simulink model "CIP_LQR_Servo"  (R2022b)
settings: Solver=ode1  StartTime=0.0  StopTime=10  FixedStep=1/1000  MaxStep=0.01  RelTol=1e-3  EnableMultiTasking=on
values from neighbouring files (symbols this model uses):
  b = [x(3) ... (first row only)    [f_inv_cart_pend.m]    (also in m_CIP_LQR_Servo.m = 0.5)
  c = 0.5    [m_CIP_LQR_Servo.m]
  C = [1 0 0 0 ... (first row only)    [m_CIP_LQR_Servo.m]
  Cp = [1 0 0 0]    [m_CIP_LQR_Servo.m]
  Cr = [0 1 0 0;0 0 1 0;0 0 0 1]    [m_CIP_LQR_Servo.m]
  D = [0;0]    [m_CIP_LQR_Servo.m]
  g = 9.81    [m_CIP_LQR_Servo.m]
  gr = GG(:,3:5)    [m_CIP_LQR_Servo.m]
  gy = GG(:,2)    [m_CIP_LQR_Servo.m]
  gz = GG(:,1)    [m_CIP_LQR_Servo.m]
  H = C    [m_CIP_LQR_Servo.m]
  k = 0    [m_CIP_LQR_Servo.m]
  L = 2    [m_CIP_LQR_Servo.m]
  M = length(f0)    [f_inv_cart_pend_jacobian_complex_step.m]    (also in m_CIP_LQR_Servo.m = 5)
  m = 1    [m_CIP_LQR_Servo.m]
  Q = diag([1e-5 1e-5 1e-8 1e-8])    [m_CIP_LQR_Servo.m]
  R = diag([1e-2 1e-2])    [m_CIP_LQR_Servo.m]
  Ts = 1/Fs    (= 0.001)    [m_CIP_LQR_Servo.m]
undefined symbols (not defined in the file or in its folder): DiscIntNeverNeededParam
libraries: aerolibanimutils x1, vrlib x1, simulink_extras x1
settings Model: Creator=ocifdaloz  LastModifiedBy=ugur
settings SolverCC: AlgebraicLoopSolver=TrustRegion
settings DataIOCC: SaveFormat=Array  SaveOutput=off  SignalLogging=off  DSMLogging=off  SaveTime=off  ReturnWorkspaceOutputs=off
settings OptimizationCC: LifeSpan=inf
settings DebuggingCC: ParameterPrecisionLossMsg=none  UnconnectedInputMsg=warning  UnconnectedOutputMsg=warning  UnconnectedLineMsg=warning  SFUnexpectedBacktrackingDiag=warning  SFNoUnconditionalDefaultTransitionDiag=warning  SFMachineParentedDataDiag=warning  ArithmeticOperatorsInVariantConditions=warning
settings HardwareCC: ProdBitPerPointer=32  ProdBitPerSizeT=32  ProdBitPerPtrDiffT=32  ProdLargestAtomicFloat=None  ProdIntDivRoundTo=Undefined  ProdEndianess=Unspecified  ProdWordSize=32  ProdHWDeviceType=32-bit Generic
settings ModelReferenceCC: EnableRefExpFcnMdlSchedulingChecks=on  PropagateSignalLabelsOutOfModel=off
settings SFSimCC: SimUseLocalCustomCode=off  CustomCodeUndefinedFunction=UseInterfaceOnly
settings RTWCC: RTWUseLocalCustomCode=off
settings CodeAppCC: StateflowObjectComments=on
settings GRTTargetCC: TargetLangStandard=C89/C90 (ANSI)
settings ConfigComp: CovMetricSettings=dw  CovSaveCumulativeToWorkspaceVar=on  CovSaveSingleToWorkspaceVar=on  CovExternalEMLEnable=off

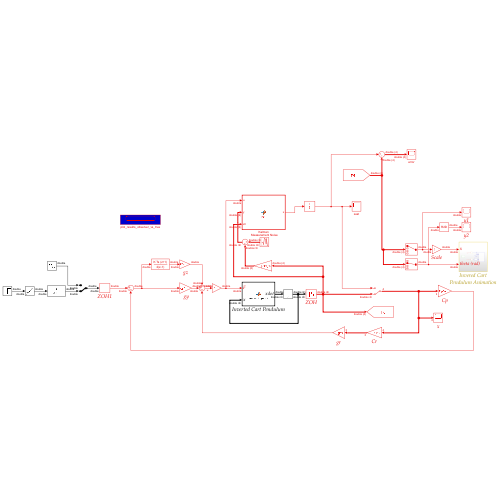
[thumbnail: Simulink's stored preview of the top-level diagram]
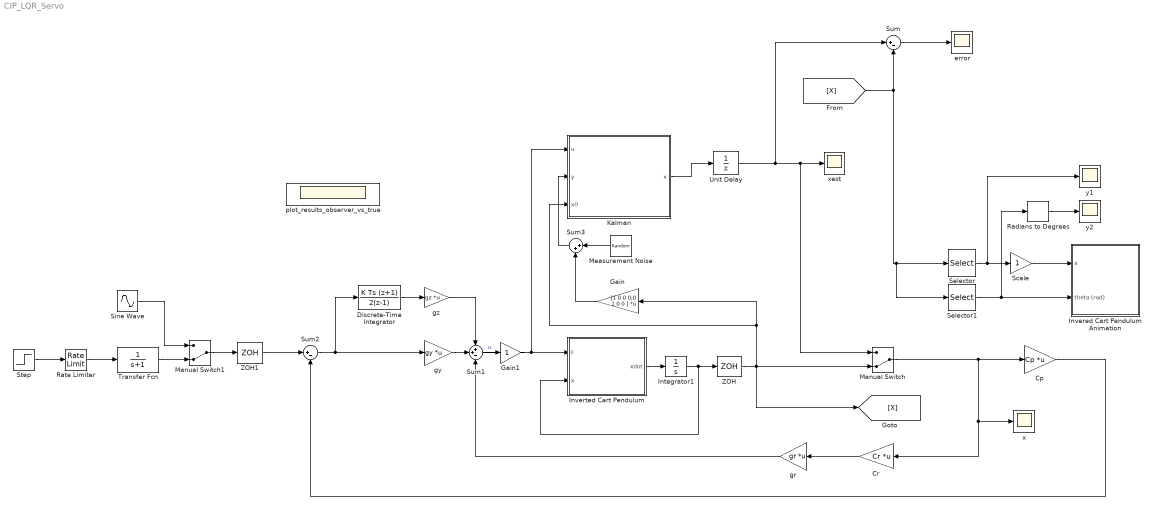
== system CIP_LQR_Servo ==
  " gy" : Gain  Gain=gy  Multiplication=Matrix(K*u)
  " gz" : Gain  Gain=gz  Multiplication=Matrix(K*u)
  Cp : Gain  Gain=Cp  Multiplication=Matrix(K*u)
  Cr : Gain  Gain=Cr  Multiplication=Matrix(K*u)
  Discrete-Time Integrator : DiscreteIntegrator  IntegratorMethod=Integration: Trapezoidal  SampleTime=Ts  ICPrevOutput=DiscIntNeverNeededParam  ICPrevScaledInput=DiscIntNeverNeededParam
  Gain : Gain  Gain=[1 0 0 0;0 1 0 0 ]  Multiplication=Matrix(K*u)
  Gain1 : Gain
  Integrator1 : Integrator  InitialCondition=[0;1*pi/180;0;0]
  Invered Cart Pendulum Animation : Subsystem
  Inverted Cart Pendulum : MATLAB Function  TreatAsAtomicUnit=on
  Kalman : MATLAB Function  TreatAsAtomicUnit=on
  Manual Switch : ManualSwitch  CurrentSetting=0
  Manual Switch1 : ManualSwitch  CurrentSetting=0
  Measurement Noise : RandomNumber  Variance=[0.01;0.01]  SampleTime=Ts
  Radians to Degrees : simulink_extras/Transformations/Radians to Degrees
  Rate Limiter : RateLimiter  SampleTimeMode=inherited
  Scale : Gain
  Selector : Selector  InputPortWidth=4  IndexOptions=Index vector (dialog)  Indices=[1]  OutputSizes=1
  Selector1 : Selector  InputPortWidth=4  IndexOptions=Index vector (dialog)  Indices=[2]  OutputSizes=1
  Sine Wave : Sin  Amplitude=45*pi/180  Frequency=2*pi*0.1  SampleTime=0
  Step : Step  Time=0  After=2  SampleTime=0
  Sum : Sum  Inputs=|+-
  Sum1 : Sum  Inputs=++-
  Sum2 : Sum  Inputs=|+-
  Sum3 : Sum  Inputs=|++
  Transfer Fcn : TransferFcn  Denominator=[1 1]
  Unit Delay : UnitDelay  SampleTime=-1  HasFrameUpgradeWarning=on
  ZOH : ZeroOrderHold  SampleTime=Ts
  ZOH1 : ZeroOrderHold  SampleTime=Ts
  error : Scope
  gr : Gain  Gain=gr  Multiplication=Matrix(K*u)
  plot_results_observer_vs_true : Scope
      settings: OpenFcn=plot_results_observer_vs_true  Floating=on
  x : Scope
  xest : Scope
  y1 : Scope
  y2 : Scope
  wires:
  Inverted Cart Pendulum/1(xdot) -> Integrator1/1
  Cp/1 -> Sum2/2
  Scale/1 -> Invered Cart Pendulum Animation/1(x)
  Selector/1 -> y1/1, Scale/1
  Sum1/1 -> Gain1/1  "u"
  Cr/1 -> gr/1
  gr/1 -> Sum1/3
  Sum2/1 -> Discrete-Time Integrator/1, " gy"/1
  " gy"/1 -> Sum1/2
  " gz"/1 -> Sum1/1
  Discrete-Time Integrator/1 -> " gz"/1
  Step/1 -> Rate Limiter/1
  Sine Wave/1 -> Manual Switch1/1
  Manual Switch1/1 -> ZOH1/1
  Radians to Degrees/1 -> y2/1
  Selector1/1 -> Radians to Degrees/1, Invered Cart Pendulum Animation/2(theta (rad))
  Transfer Fcn/1 -> Manual Switch1/2
  Rate Limiter/1 -> Transfer Fcn/1
  ZOH1/1 -> Sum2/1
  Sum/1 -> error/1
  ZOH/1 -> Manual Switch/2, [X], Kalman/3(x0), Gain/1
  Manual Switch/1 -> Cr/1, x/1, Cp/1
  Integrator1/1 -> Inverted Cart Pendulum/2(x), ZOH/1
  [X] -> Selector1/1, Selector/1, Sum/2
  Kalman/1(x) -> Unit Delay/1
  Unit Delay/1 -> xest/1, Manual Switch/1, Sum/1
  Measurement Noise/1 -> Sum3/1
  Sum3/1 -> Kalman/2(y)
  Gain/1 -> Sum3/2
  Gain1/1 -> Kalman/1(u), Inverted Cart Pendulum/1(F)

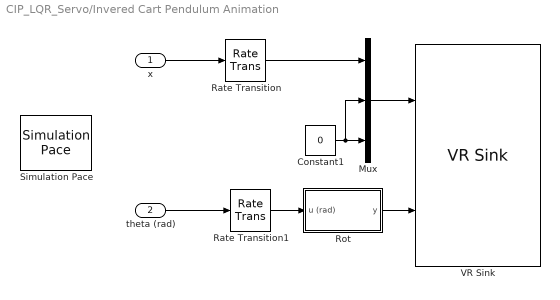
== system CIP_LQR_Servo/Invered Cart Pendulum Animation ==
  x : Inport
  theta (rad) : Inport  Port=2
  Constant1 : Constant  Value=0  SampleTime=-1
  Mux : Mux  Inputs=3
  Rate Transition : RateTransition  OutPortSampleTime=0.1
  Rate Transition1 : RateTransition  OutPortSampleTime=0.1
  Rot : Subsystem
  Simulation Pace : aerolibanimutils/Simulation Pace  SimulationPace=1  SleepMode=Auto  OutputPaceError=off  SampleTime=1/20
  VR Sink : vrlib/VR Sink  InstantiateOnLoad=on  SampleTime=0.1  ViewEnable=on  RemoteChange=off  RemoteView=off  FieldsWritten=Cart_Frame.translation.3.1.1.double#Pendulum_Frame.rotation.4.1.1.double  WorldFileName=Inv_Cart_Pendulum.wrl  AutoView=off  VideoDimensions=[]  AllowVariableSize=off
  wires:
  theta (rad)/1 -> Rate Transition1/1
  Constant1/1 -> Mux/2, Mux/3
  x/1 -> Rate Transition/1
  Rate Transition/1 -> Mux/1
  Rate Transition1/1 -> Rot/1(u (rad))
  Mux/1 -> VR Sink/1
  Rot/1(y) -> VR Sink/2

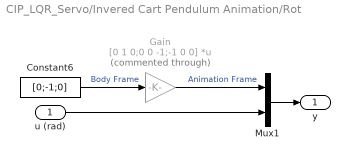
== system CIP_LQR_Servo/Invered Cart Pendulum Animation/Rot ==
  u (rad) : Inport
  Constant6 : Constant  Value=[0;-1;0]  SampleTime=-1
  Gain : Gain  Commented=through  Gain=[0 1 0;0 0 -1;-1 0 0]  Multiplication=Matrix(K*u)
  Mux1 : Mux  Inputs=2
  y : Outport  VectorParamsAs1DForOutWhenUnconnected=off
  wires:
  Constant6/1 -> Gain/1  "Body Frame"
  Gain/1 -> Mux1/1  "Animation Frame"
  u (rad)/1 -> Mux1/2
  Mux1/1 -> y/1

== matlab function CIP_LQR_Servo/Kalman ==
  data: u input; x output; y input; H parameter; Q parameter; R parameter; M parameter; m parameter; L parameter; g parameter; c parameter; b parameter; k parameter; C parameter; D parameter; Ts parameter; x0 input
function x = fcn(u,y,H,Q,R,M, m, L, g, c, b, k,C, D,Ts,x0)

persistent xest_before P_before
if isempty(xest_before)
    xest_before=zeros(4,1);
    P_before=eye(4);
end

[F,G]=getsvalue(x0,u,M,m,L, g, c, b, k,C,D,Ts);

%Predict
xest=F*xest_before+G*u;
Pest=F*P_before*F'+Q;

%Update
y_error=y-H*xest;
Sk=H*Pest*H'+R;
Kk=Pest*H'*inv(Sk);
x=xest+Kk*y_error;
P=(eye(4)-Kk*H)*Pest;
% y_error=y-H*x;

P_before=P;
xest_before=x;
end

== matlab function CIP_LQR_Servo/Inverted Cart Pendulum ==
  data: F input; x input; xdot output; M parameter size=1; m parameter size=1; L parameter size=1; g parameter size=1; c parameter size=1; b parameter size=1; k parameter
function xdot = inv_cart_pend(F, x, M, m, L, g, c, b, k)
%#codege
 
xdot=f_inv_cart_pend(x, F, M, m, L, g, c, b, k);
